simulink model "Lab1_printer"  (R2019b)
settings: Solver=VariableStepAuto  StartTime=0.0  StopTime=100  RelTol=1e-3
undefined symbols (not defined in the file): DiscIntNeverNeededParam
libraries: simulink x1
settings Model: Creator=Siemen  LastModifiedBy=Siemen

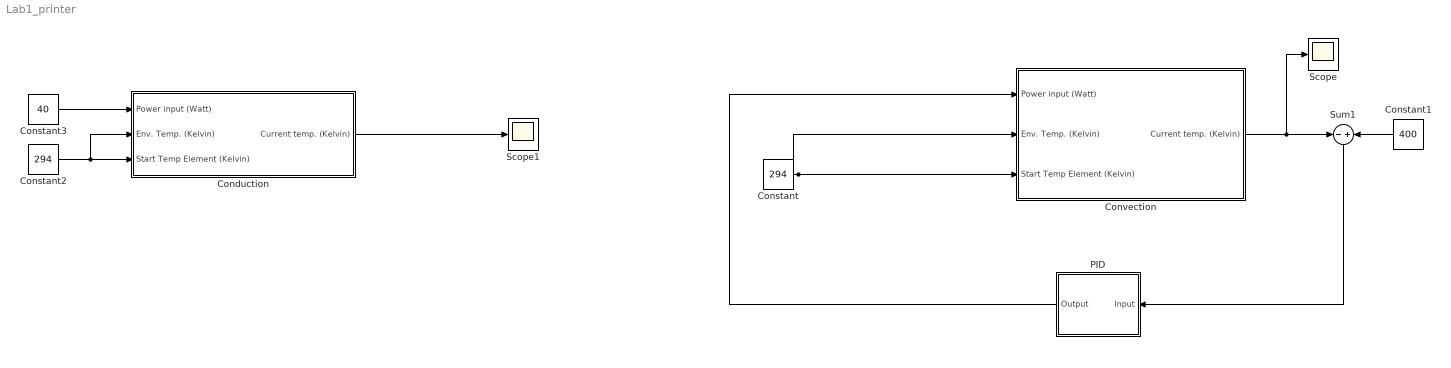
== system Lab1_printer ==
  "Conduction " : Subsystem
  Constant : Constant  Value=294
  Constant1 : Constant  Value=400
  Constant2 : Constant  Value=294
  Constant3 : Constant  Value=40
  Convection : Subsystem
  PID : Subsystem  TreatAsAtomicUnit=on  SystemSampleTime=0.1
  Scope : Scope
  Scope1 : Scope
  Sum1 : Sum  Inputs=-+
  wires:
  Constant/1 -> Convection/2(Env. Temp. (Kelvin)), Convection/3(Start Temp Element (Kelvin))
  "Conduction "/1("Current temp. (Kelvin) ") -> Scope1/1
  Constant2/1 -> "Conduction "/2(Env. Temp. (Kelvin)), "Conduction "/3(Start Temp Element (Kelvin))
  Constant3/1 -> "Conduction "/1("Power input (Watt) ")
  Convection/1(Current temp. (Kelvin)) -> Scope/1, Sum1/1
  Constant1/1 -> Sum1/2
  Sum1/1 -> PID/1(Input)
  PID/1(Output) -> Convection/1(Power input (Watt))

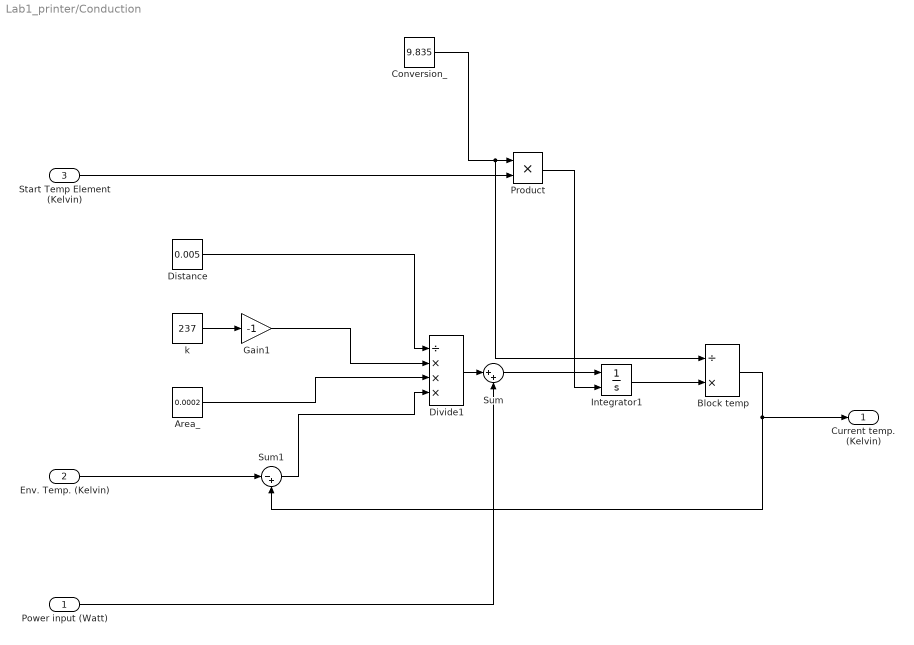
== system Lab1_printer/Conduction  ==
  "Power input (Watt) " : Inport
  Env. Temp. (Kelvin) : Inport  Port=2
  Start Temp Element (Kelvin) : Inport  Port=3
  Area_ : Constant  Value=0.0002
  "Block temp " : Product  Inputs=/*
  Conversion_ : Constant  Value=9.835
  Distance : Constant  Value=0.005
  Divide1 : Product  Inputs=/***
  Gain1 : Gain  Gain=-1
  Integrator1 : Integrator  InitialConditionSource=external
  Product : Product
  Sum : Sum  Inputs=|++
  Sum1 : Sum  Inputs=|-+
  "k " : Constant  Value=237
  "Current temp. (Kelvin) " : Outport
  wires:
  Product/1 -> Integrator1/2
  Sum1/1 -> Divide1/4
  Conversion_/1 -> Product/1, "Block temp "/1
  Divide1/1 -> Sum/1
  Integrator1/1 -> "Block temp "/2
  Distance/1 -> Divide1/1
  Start Temp Element (Kelvin)/1 -> Product/2
  "Power input (Watt) "/1 -> Sum/2
  Sum/1 -> Integrator1/1
  Gain1/1 -> Divide1/2
  Env. Temp. (Kelvin)/1 -> Sum1/1
  "Block temp "/1 -> "Current temp. (Kelvin) "/1, Sum1/2
  Area_/1 -> Divide1/3
  "k "/1 -> Gain1/1

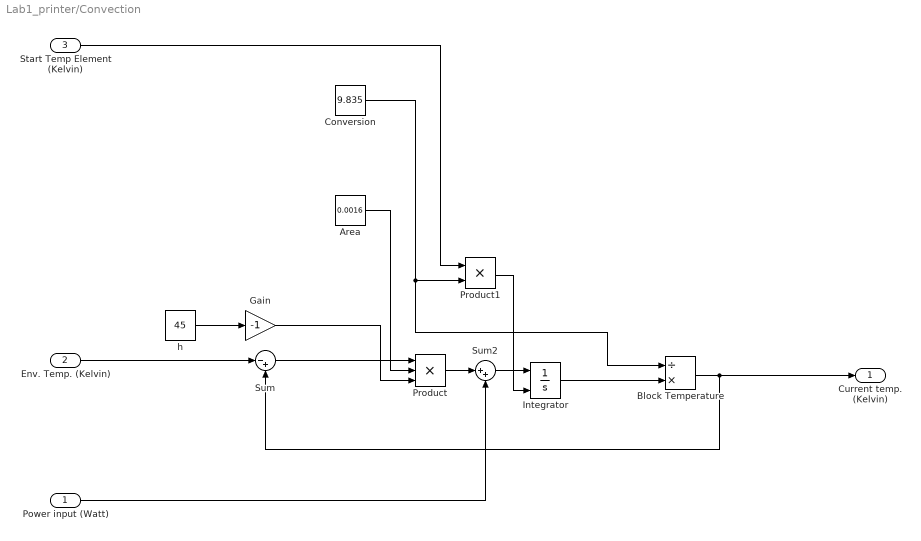
== system Lab1_printer/Convection ==
  Power input (Watt) : Inport
  Env. Temp. (Kelvin) : Inport  Port=2
  Start Temp Element (Kelvin) : Inport  Port=3
  "Area " : Constant  Description=area  Value=0.0016
  "Block Temperature " : Product  Inputs=/*
  Conversion : Constant  Value=9.835
  Gain : Gain  Gain=-1
  Integrator : Integrator  InitialConditionSource=external
  Product : Product  Inputs=3
  Product1 : Product
  Sum : Sum  Inputs=|-+
  Sum2 : Sum  Inputs=|++
  h : Constant  Description=h: heat transfer coefficient  Value=45
  Current temp. (Kelvin) : Outport
  wires:
  Integrator/1 -> "Block Temperature "/2
  Sum2/1 -> Integrator/1
  Start Temp Element (Kelvin)/1 -> Product1/1
  "Area "/1 -> Product/2
  Sum/1 -> Product/1
  Product/1 -> Sum2/1
  Conversion/1 -> "Block Temperature "/1, Product1/2
  Power input (Watt)/1 -> Sum2/2
  "Block Temperature "/1 -> Sum/2, Current temp. (Kelvin)/1
  Product1/1 -> Integrator/2
  Env. Temp. (Kelvin)/1 -> Sum/1
  h/1 -> Gain/1
  Gain/1 -> Product/3

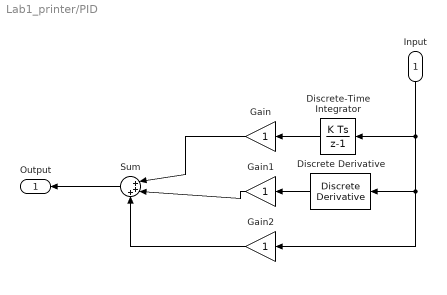
== system Lab1_printer/PID ==
  Input : Inport
  Discrete Derivative : simulink/Discrete/Discrete Derivative  gainval=1.0  ICPrevScaledInput=0.0  OutMin=[]  OutMax=[]  OutDataType=fixdt(1, 16)  OutScaling=2^-10  DoSatur=off
  Discrete-Time Integrator : DiscreteIntegrator  SampleTime=-1  ICPrevOutput=DiscIntNeverNeededParam  ICPrevScaledInput=DiscIntNeverNeededParam
  Gain : Gain
  Gain1 : Gain
  Gain2 : Gain
  Sum : Sum  Inputs=|+++
  Output : Outport
  wires:
  Gain/1 -> Sum/1
  Gain2/1 -> Sum/3
  Sum/1 -> Output/1
  Discrete Derivative/1 -> Gain1/1
  Input/1 -> Discrete-Time Integrator/1, Discrete Derivative/1, Gain2/1
  Gain1/1 -> Sum/2
  Discrete-Time Integrator/1 -> Gain/1
